simulink library "calcAeroCoeffs2_cl"  (R2020a)
settings: Solver=VariableStepAuto  StartTime=0.0  StopTime=10.0  RelTol=1e-3
settings Model: Creator=Ayaz  LastModifiedBy=Ayaz

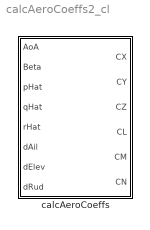
== system calcAeroCoeffs2_cl ==
  calcAeroCoeffs : Subsystem

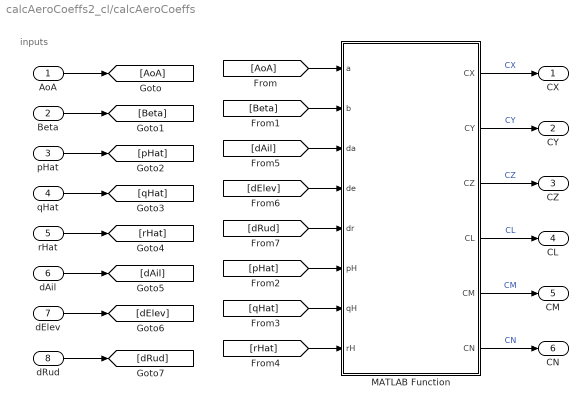
== system calcAeroCoeffs2_cl/calcAeroCoeffs ==
  note: inputs
  AoA : Inport
  Beta : Inport  Port=2
  pHat : Inport  Port=3
  qHat : Inport  Port=4
  rHat : Inport  Port=5
  dAil : Inport  Port=6
  dElev : Inport  Port=7
  dRud : Inport  Port=8
  MATLAB Function : MATLAB Function  TreatAsAtomicUnit=on
  CX : Outport
  CY : Outport  Port=2
  CZ : Outport  Port=3
  CL : Outport  Port=4
  CM : Outport  Port=5
  CN : Outport  Port=6
  wires:
  AoA/1 -> [AoA]
  Beta/1 -> [Beta]
  pHat/1 -> [pHat]
  qHat/1 -> [qHat]
  rHat/1 -> [rHat]
  dAil/1 -> [dAil]
  dElev/1 -> [dElev]
  dRud/1 -> [dRud]
  [AoA] -> MATLAB Function/1(a)
  [Beta] -> MATLAB Function/2(b)
  [pHat] -> MATLAB Function/6(pH)
  [qHat] -> MATLAB Function/7(qH)
  [rHat] -> MATLAB Function/8(rH)
  [dAil] -> MATLAB Function/3(da)
  [dElev] -> MATLAB Function/4(de)
  [dRud] -> MATLAB Function/5(dr)
  MATLAB Function/1(CX) -> CX/1  "CX"
  MATLAB Function/2(CY) -> CY/1  "CY"
  MATLAB Function/3(CZ) -> CZ/1  "CZ"
  MATLAB Function/4(CL) -> CL/1  "CL"
  MATLAB Function/5(CM) -> CM/1  "CM"
  MATLAB Function/6(CN) -> CN/1  "CN"

== matlab function calcAeroCoeffs2_cl/calcAeroCoeffs/MATLAB Function ==
  data: a input; CX output; b input; da input; de input; dr input; pH input; qH input; rH input; CY output; CZ output; CL output; CM output; CN output
function [CX,CY,CZ,CL,CM,CN] = calculateAeroCoeff(a,b,da,de,dr,pH,qH,rH)

[CX,CY,CZ,CL,CM,CN] = calculateAeroCoeff(a,b,da,de,dr,pH,qH,rH);

end
